simulink model "diffdriveLQR"  (R2020b)
settings: Solver=VariableStepAuto  StartTime=0.0  StopTime=100  RelTol=1e-3
undefined symbols (not defined in the file): LQR
libraries: pid_lib x1
settings Model: Creator=Kevin  LastModifiedBy=Kevin

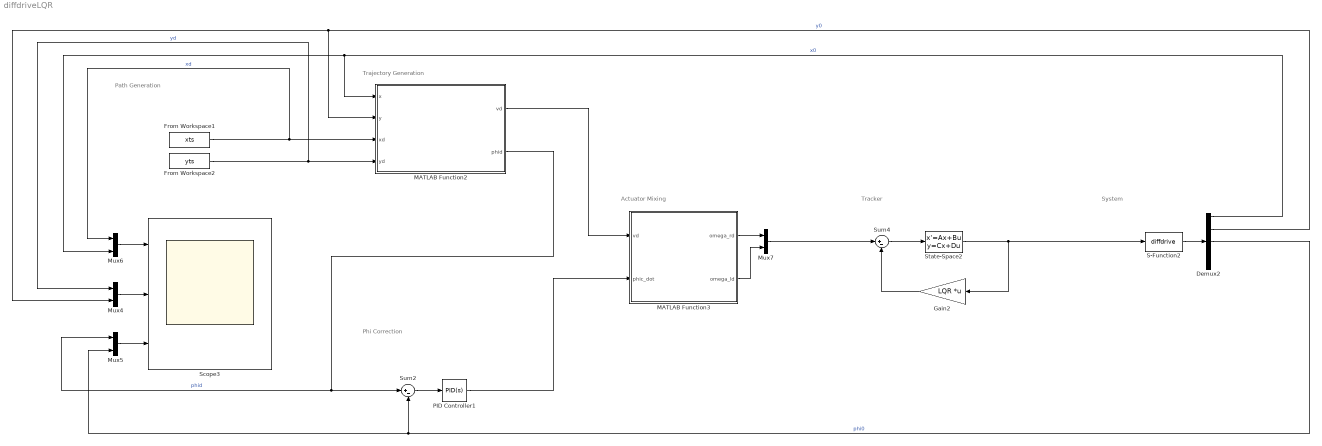
== system diffdriveLQR ==
  note: Phi Correction
  note: Trajectory Generation
  note: Actuator Mixing
  note: Tracker
  note: System
  note: Path Generation
  Demux2 : Demux  Outputs=5
  From Workspace1 : FromWorkspace  VariableName=xts
  From Workspace2 : FromWorkspace  VariableName=yts
  Gain2 : Gain  Gain=LQR  Multiplication=Matrix(K*u)
  MATLAB Function2 : MATLAB Function  TreatAsAtomicUnit=on
  MATLAB Function3 : MATLAB Function  TreatAsAtomicUnit=on
  Mux{4..7} (4 alike) : Mux  Inputs=2
  PID Controller1 : pid_lib/PID Controller  Controller=PID  Form=Parallel  TimeDomain=Continuous-time  UseExternalTs=off  SampleTime=-1  IntegratorMethod=Forward Euler  FilterMethod=Forward Euler  ControllerParametersSource=internal  P=-35.3272819098551  I=-52.2325684390587  D=-2.60564792973815  UseFilter=on  N=1915.34348084941  TunerSelectOption=Transfer Function Based (PID Tuner App)  InitialConditionSource=internal  InitialConditionForIntegrator=0  InitialConditionForFilter=0  DifferentiatorICPrevScaledInput=0  ExternalReset=none  TrackingMode=off  Kt=1  LimitOutput=off  SatLimitsSource=internal  UpperSaturationLimit=inf  LowerSaturationLimit=-inf  LinearizeAsGain=on  AntiWindupMode=none  Kb=1  POutMin=[]  POutMax=[]  IOutMin=[]  IOutMax=[]  DOutMin=[]  DOutMax=[]  NOutMin=[]  NOutMax=[]  SumOutMin=[]  SumOutMax=[]  SaturationOutMin=[]  SaturationOutMax=[]  PParamMin=[]  PParamMax=[]  IParamMin=[]  IParamMax=[]  DParamMin=[]  DParamMax=[]  NParamMin=[]  NParamMax=[]  KbParamMin=[]  KbParamMax=[]  KtParamMin=[]  KtParamMax=[]  KbOutMin=[]  KbOutMax=[]  KtOutMin=[]  KtOutMax=[]  IntegratorOutMin=[]  IntegratorOutMax=[]  FilterOutMin=[]  FilterOutMax=[]  SumI1OutMin=[]  SumI1OutMax=[]  SumI2OutMin=[]  SumI2OutMax=[]  SumI3OutMin=[]  SumI3OutMax=[]  SumI4OutMin=[]  SumI4OutMax=[]  SumDOutMin=[]  SumDOutMax=[]  DifferentiatorOutMin=[]  DifferentiatorOutMax=[]  FilterDiffOutCoefMin=[]  FilterDiffOutCoefMax=[]  ReciprocalOutMin=[]  ReciprocalOutMax=[]  SumDenOutMin=[]  SumDenOutMax=[]  SumNumOutMin=[]  SumNumOutMax=[]  DivideOutMin=[]  DivideOutMax=[]  UdiffTsProdOutMin=[]  UdiffTsProdOutMax=[]  NTsProdOutMin=[]  NTsProdOutMax=[]  UintegralTsProdOutMin=[]  UintegralTsProdOutMax=[]  UngainTsProdOutMin=[]  UngainTsProdOutMax=[]  IntegratorContinuousStateAttributes=''  IntegratorStateMustResolveToSignalObject=off  IntegratorRTWStateStorageClass=Auto  FilterContinuousStateAttributes=''  FilterStateMustResolveToSignalObject=off  FilterRTWStateStorageClass=Auto  ParallelPVariant=InternalParameters  IdealPVariant=Disabled  IVariant=InternalParameters  DVariant=InternalParameters  IntegratorVariant=Continuous  SatVariant=Disabled  AWVariant=Passthrough  PCopyVariant=Disabled  TRVariant=Disabled  FdbkBlocksVariant=Forward  IdealPFdbkVariant=Disabled  SatFdbkVariant=Disabled  DerivativeFilterVariant=ContFilter  NVariant=InternalParameters  NCopyVariant=Disabled  FilterICVariant=InternalICsFilter  IntegratorICVariant=InternalICs  ExternalResetVariant=Disabled  TRSumVariant=Passthrough  SumFdbkVariant=Disabled  SumVariant=Sum_PID  TsampFilterVariant=InternalTs  TsampNgainVariant=Passthrough  TsampIntegralVariant=Passthrough  ExternalSaturationOutDataTypeStr=Inherit: Same as second input
  S-Function2 : S-Function  FunctionName=diffdrive  SFunctionDeploymentMode=off  EnableBusSupport=off
  Scope3 : Scope  NumInputPorts=3
  State-Space2 : StateSpace  A=[-10.3 0; 0 -9.4318]  B=[30 0; 0 26.5152]  C=[1 0; 0 1]  D=[0 0; 0 0]  InitialCondition=0
  Sum2 : Sum  Inputs=|+-
  Sum4 : Sum  Inputs=|+-
  wires:
  State-Space2/1 -> S-Function2/1, Gain2/1
  Gain2/1 -> Sum4/2
  MATLAB Function3/1(omega_rd) -> Mux7/1
  MATLAB Function3/2(omega_ld) -> Mux7/2
  S-Function2/1 -> Demux2/1
  From Workspace1/1 -> Mux6/1, MATLAB Function2/3(xd)  "xd"
  From Workspace2/1 -> Mux4/1, MATLAB Function2/4(yd)  "yd"
  MATLAB Function2/1(vd) -> MATLAB Function3/1(vd)
  MATLAB Function2/2(phid) -> Sum2/1, Mux5/1  "phid"
  PID Controller1/1 -> MATLAB Function3/2(phic_dot)
  Demux2/3 -> Sum2/2, Mux5/2  "phi0"
  Demux2/2 -> MATLAB Function2/2(y), Mux4/2  "y0"
  Demux2/1 -> Mux6/2, MATLAB Function2/1(x)  "x0"
  Mux6/1 -> Scope3/1
  Mux4/1 -> Scope3/2
  Mux5/1 -> Scope3/3
  Mux7/1 -> Sum4/1
  Sum2/1 -> PID Controller1/1
  Sum4/1 -> State-Space2/1

== matlab function diffdriveLQR/MATLAB Function2 ==
  data: x input; y input; xd input; vd output; yd input; phid output
function [vd,phid] = TrajectoryGeneration(x,y,xd,yd)

% velocity gain between 0 and 1
% chosen to be 0.5 as a good median
alpha = 0.5;

% calculation of phid and vd with error checking for NaN
if isnan(atan((yd-y)/(xd-x)))
    phid = 0;
else
    phid = atan((yd-y)/(xd-x));
end

if isnan(alpha*sqrt(((xd-x)^2)+((yd-y)^2)))
    vd = 0;
else
    vd = alpha*sqrt(((xd-x)^2)+((yd-y)^2));
end

== matlab function diffdriveLQR/MATLAB Function3 ==
  data: vd input; omega_rd output; omega_ld output; phic_dot input
function [omega_rd,omega_ld] = ActuatorMixing(vd,phic_dot)

% radius of the wheel
r=2;
% half the distance between the driven wheels
d=4;

% convert from (vd, phic_dot) to (omega_rd, omega_ld)
omega_rd = ((2*vd)+(phic_dot*d))/(2*r);
omega_ld = ((2*vd)-(phic_dot*d))/(2*r);
